simulink model "skyhookMRcontrol"  (R2016a)
settings: Solver=VariableStepAuto  StartTime=0.0  StopTime=10.0  RelTol=1e-3
undefined symbols (not defined in the file): b1, k1, k2, m1, m2
libraries: simulink x1
settings Model: Creator=mm395  LastModifiedBy=mm395

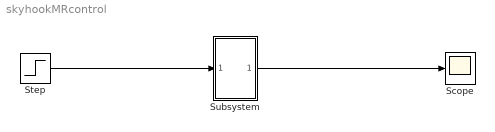
== system skyhookMRcontrol ==
  Scope : Scope
  Step : Step  SampleTime=0  ZeroCross=off
  Subsystem : Subsystem
  wires:
  Subsystem/1(Out1) -> Scope/1
  Step/1 -> Subsystem/1(In1)

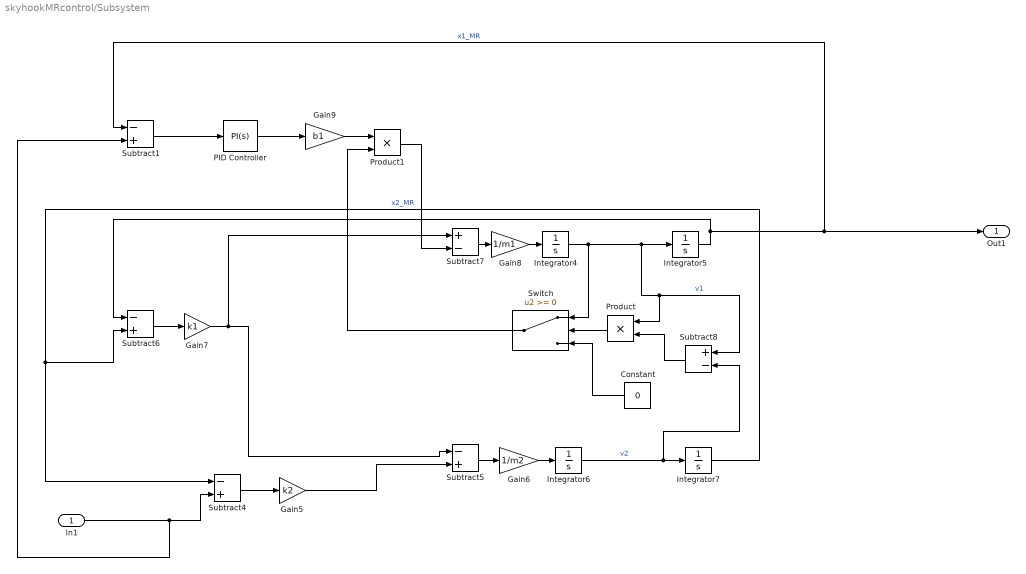
== system skyhookMRcontrol/Subsystem ==
  In1 : Inport
  Constant : Constant  Value=0
  Gain5 : Gain  Gain=k2
  Gain6 : Gain  Gain=1/m2
  Gain7 : Gain  Gain=k1
  Gain8 : Gain  Gain=1/m1
  Gain9 : Gain  Gain=b1
  Integrator{4..7} (4 alike) : Integrator
  PID Controller : simulink/Continuous/PID Controller  Controller=PI  TimeDomain=Continuous-time  SampleTime=-1  IntegratorMethod=Forward Euler  FilterMethod=Forward Euler  Form=Parallel  UseFilter=on  ControllerParametersSource=internal  P=0  I=-1  D=0  N=100  InitialConditionSource=internal  InitialConditionForIntegrator=0  InitialConditionForFilter=0  ExternalReset=none  LimitOutput=off  UpperSaturationLimit=inf  LowerSaturationLimit=-inf  LinearizeAsGain=on  AntiWindupMode=none  Kb=1  TrackingMode=off  Kt=1  PParamMin=[]  PParamMax=[]  IParamMin=[]  IParamMax=[]  DParamMin=[]  DParamMax=[]  NParamMin=[]  NParamMax=[]  KbParamMin=[]  KbParamMax=[]  KtParamMin=[]  KtParamMax=[]  POutMin=[]  POutMax=[]  IOutMin=[]  IOutMax=[]  DOutMin=[]  DOutMax=[]  NOutMin=[]  NOutMax=[]  KbOutMin=[]  KbOutMax=[]  KtOutMin=[]  KtOutMax=[]  IntegratorOutMin=[]  IntegratorOutMax=[]  FilterOutMin=[]  FilterOutMax=[]  SumOutMin=[]  SumOutMax=[]  SumI1OutMin=[]  SumI1OutMax=[]  SumI2OutMin=[]  SumI2OutMax=[]  SumI3OutMin=[]  SumI3OutMax=[]  SumDOutMin=[]  SumDOutMax=[]  SaturationOutMin=[]  SaturationOutMax=[]  IntegratorContinuousStateAttributes=''  IntegratorStateMustResolveToSignalObject=off  IntegratorRTWStateStorageClass=Auto  FilterContinuousStateAttributes=''  FilterStateMustResolveToSignalObject=off  FilterRTWStateStorageClass=Auto  DifferentiatorICPrevScaledInput=0  DifferentiatorOutMin=[]  DifferentiatorOutMax=[]
  Product : Product
  Product1 : Product
  Subtract{1,4..6} (4 alike) : Sum  Inputs=-+
  Subtract7 : Sum  Inputs=+-
  Subtract8 : Sum  Inputs=+-
  Switch : Switch  ZeroCross=off
  Out1 : Outport
  wires:
  Switch/1 -> Product1/2
  Gain9/1 -> Product1/1
  Subtract7/1 -> Gain8/1
  Product/1 -> Switch/2
  Gain7/1 -> Subtract5/1, Subtract7/1
  Subtract6/1 -> Gain7/1
  Integrator4/1 -> Switch/1, Integrator5/1, Subtract8/1, Product/1  "v1"
  Gain8/1 -> Integrator4/1
  Subtract8/1 -> Product/2
  Gain5/1 -> Subtract5/2
  Subtract4/1 -> Gain5/1
  Integrator7/1 -> Subtract6/2, Subtract4/1  "x2_MR"
  Integrator6/1 -> Subtract8/2, Integrator7/1  "v2"
  Gain6/1 -> Integrator6/1
  Subtract5/1 -> Gain6/1
  Constant/1 -> Switch/3
  Integrator5/1 -> Subtract6/1, Out1/1, Subtract1/1  "x1_MR"
  Product1/1 -> Subtract7/2
  In1/1 -> Subtract4/2, Subtract1/2
  Subtract1/1 -> PID Controller/1
  PID Controller/1 -> Gain9/1
